simulink model "lineOverBlocks"  (R2016b)
settings: Solver=VariableStepAuto  StartTime=0.0  StopTime=10.0  RelTol=1e-3
settings Model: Creator=Harjot  LastModifiedBy=Harjot

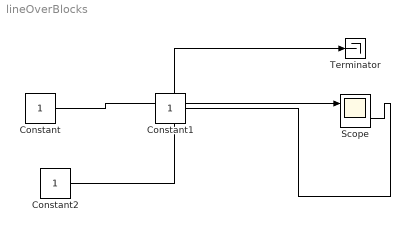
== system lineOverBlocks ==
  Constant : Constant
  Constant1 : Constant
  Constant2 : Constant
  Scope : Scope  NumInputPorts=2
  Terminator : Terminator
  wires:
  Constant1/1 -> Scope/2
  Constant/1 -> Scope/1
  Constant2/1 -> Terminator/1
